simulink model "SMC_Lyapunov_PID_switch_com_m_change"  (R2016a)
settings: Solver=VariableStepAuto  StartTime=0.0  StopTime=50  RelTol=1e-3
libraries: simulink x2
settings Model: Creator=Jie WEN  LastModifiedBy=张涵

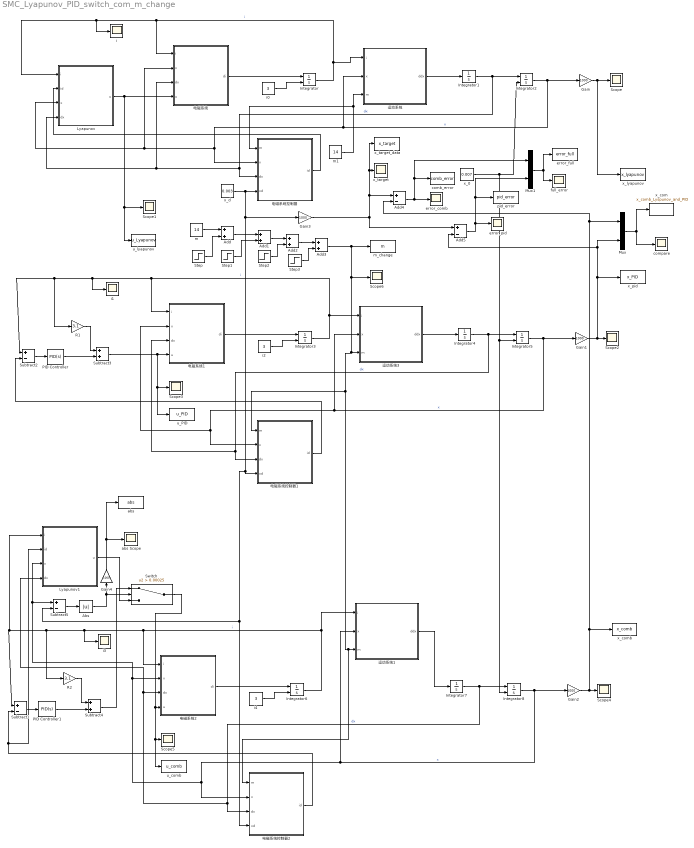
== system SMC_Lyapunov_PID_switch_com_m_change ==
  Abs : Abs
  Add{,1..3} (4 alike) : Sum
  Add4 : Sum  Inputs=+-
  Add5 : Sum  Inputs=+-
  Gain{,1..4} (5 alike) : Gain  Gain=1000
  Integrator : Integrator  InitialConditionSource=external  InitialCondition=3
  Integrator1 : Integrator
  Integrator2 : Integrator  InitialConditionSource=external  InitialCondition=7
  Integrator3 : Integrator  InitialConditionSource=external  InitialCondition=3
  Integrator4 : Integrator
  Integrator5 : Integrator  InitialConditionSource=external  InitialCondition=7
  Integrator6 : Integrator  InitialConditionSource=external  InitialCondition=3
  Integrator7 : Integrator
  Integrator8 : Integrator  InitialConditionSource=external  InitialCondition=7
  Lyapunov : MATLAB Function  TreatAsAtomicUnit=on
  Lyapunov1 : MATLAB Function  TreatAsAtomicUnit=on
  Mux : Mux  Inputs=2
  Mux1 : Mux  Inputs=2
  PID Controller : simulink/Continuous/PID Controller  Controller=PID  Form=Parallel  TimeDomain=Continuous-time  SampleTime=-1  IntegratorMethod=Forward Euler  ControllerParametersSource=internal  P=-6  I=0.1  D=0.1  UseFilter=on  N=100  InitialConditionSource=internal  InitialConditionForIntegrator=0  InitialConditionForFilter=0  DifferentiatorICPrevScaledInput=0  ExternalReset=none  TrackingMode=off  Kt=1  LimitOutput=off  UpperSaturationLimit=inf  LowerSaturationLimit=-inf  LinearizeAsGain=on  AntiWindupMode=none  Kb=1  POutMin=[]  POutMax=[]  IOutMin=[]  IOutMax=[]  DOutMin=[]  DOutMax=[]  NOutMin=[]  NOutMax=[]  SumOutMin=[]  SumOutMax=[]  SaturationOutMin=[]  SaturationOutMax=[]  PParamMin=[]  PParamMax=[]  IParamMin=[]  IParamMax=[]  DParamMin=[]  DParamMax=[]  NParamMin=[]  NParamMax=[]  KbParamMin=[]  KbParamMax=[]  KtParamMin=[]  KtParamMax=[]  KbOutMin=[]  KbOutMax=[]  KtOutMin=[]  KtOutMax=[]  IntegratorOutMin=[]  IntegratorOutMax=[]  FilterOutMin=[]  FilterOutMax=[]  SumI1OutMin=[]  SumI1OutMax=[]  SumI2OutMin=[]  SumI2OutMax=[]  SumI3OutMin=[]  SumI3OutMax=[]  SumDOutMin=[]  SumDOutMax=[]  DifferentiatorOutMin=[]  DifferentiatorOutMax=[]  IntegratorContinuousStateAttributes=''  IntegratorStateMustResolveToSignalObject=off  IntegratorRTWStateStorageClass=Auto  FilterContinuousStateAttributes=''  FilterStateMustResolveToSignalObject=off  FilterRTWStateStorageClass=Auto
  PID Controller1 : simulink/Continuous/PID Controller  Controller=PID  Form=Parallel  TimeDomain=Continuous-time  SampleTime=-1  IntegratorMethod=Forward Euler  ControllerParametersSource=internal  P=-6  I=0.1  D=0.1  UseFilter=on  N=100  InitialConditionSource=internal  InitialConditionForIntegrator=0  InitialConditionForFilter=0  DifferentiatorICPrevScaledInput=0  ExternalReset=none  TrackingMode=off  Kt=1  LimitOutput=off  UpperSaturationLimit=inf  LowerSaturationLimit=-inf  LinearizeAsGain=on  AntiWindupMode=none  Kb=1  POutMin=[]  POutMax=[]  IOutMin=[]  IOutMax=[]  DOutMin=[]  DOutMax=[]  NOutMin=[]  NOutMax=[]  SumOutMin=[]  SumOutMax=[]  SaturationOutMin=[]  SaturationOutMax=[]  PParamMin=[]  PParamMax=[]  IParamMin=[]  IParamMax=[]  DParamMin=[]  DParamMax=[]  NParamMin=[]  NParamMax=[]  KbParamMin=[]  KbParamMax=[]  KtParamMin=[]  KtParamMax=[]  KbOutMin=[]  KbOutMax=[]  KtOutMin=[]  KtOutMax=[]  IntegratorOutMin=[]  IntegratorOutMax=[]  FilterOutMin=[]  FilterOutMax=[]  SumI1OutMin=[]  SumI1OutMax=[]  SumI2OutMin=[]  SumI2OutMax=[]  SumI3OutMin=[]  SumI3OutMax=[]  SumDOutMin=[]  SumDOutMax=[]  DifferentiatorOutMin=[]  DifferentiatorOutMax=[]  IntegratorContinuousStateAttributes=''  IntegratorStateMustResolveToSignalObject=off  IntegratorRTWStateStorageClass=Auto  FilterContinuousStateAttributes=''  FilterStateMustResolveToSignalObject=off  FilterRTWStateStorageClass=Auto
  R1 : Gain  Gain=3.1
  R2 : Gain  Gain=3.1
  Scope{,1..6} (7 alike) : Scope
  Step : Step  Time=10  After=0.2  SampleTime=0
  Step1 : Step  Time=20  After=-0.2  SampleTime=0
  Step2 : Step  Time=30  After=-0.1  SampleTime=0
  Step3 : Step  Time=40  After=0.1  SampleTime=0
  Subtract1 : Sum  Inputs=+-
  Subtract2 : Sum  Inputs=+-
  Subtract3 : Sum
  Subtract4 : Sum
  Subtract5 : Sum  Inputs=+-
  Switch : Switch  Criteria=u2 > Threshold  Threshold=0.00025
  abs : ToWorkspace  VariableName=abs  SampleTime=-1
  abs Scope : Scope
  comb_error : ToWorkspace  VariableName=comb_error  SampleTime=-1
  compare : Scope
  error_comb : Scope
  error_full : ToWorkspace  VariableName=error_full  SampleTime=-1
  error_pid : Scope
  full_error : Scope
  i : Scope
  i0 : Constant  Value=3
  i1 : Scope
  i2 : Constant  Value=3
  i3 : Scope
  i4 : Constant  Value=3
  m : Constant  Value=14
  m1 : Constant  Value=14
  m_change : ToWorkspace  VariableName=m  SampleTime=-1
  pid_error : ToWorkspace  VariableName=pid_error  SampleTime=-1
  u_PID : ToWorkspace  VariableName=u_PID  SampleTime=-1
  u_comb : ToWorkspace  VariableName=u_comb  SampleTime=-1
  u_lyapunov : ToWorkspace  VariableName=u_Lyapunov  SampleTime=-1
  x_0 : Constant  Value=0.007
  x_com : ToWorkspace  VariableName=x_comb_Lyspunov_and_PID  SampleTime=-1
  x_comb : ToWorkspace  VariableName=x_comb  SampleTime=-1
  x_d : Constant  Value=0.003
  x_lyapunov : ToWorkspace  VariableName=x_lyapunov  SampleTime=-1
  x_pid : ToWorkspace  VariableName=x_PID  SampleTime=-1
  x_target : Scope
  x_target_data : ToWorkspace  VariableName=x_target  SampleTime=-1
  电磁系统 : MATLAB Function  TreatAsAtomicUnit=on
  电磁系统1 : MATLAB Function  TreatAsAtomicUnit=on
  电磁系统2 : MATLAB Function  TreatAsAtomicUnit=on
  电磁系统控制器 : MATLAB Function  TreatAsAtomicUnit=on
  电磁系统控制器1 : MATLAB Function  TreatAsAtomicUnit=on
  电磁系统控制器2 : MATLAB Function  TreatAsAtomicUnit=on
  运动系统 : MATLAB Function  TreatAsAtomicUnit=on
  运动系统1 : MATLAB Function  TreatAsAtomicUnit=on
  运动系统3 : MATLAB Function  TreatAsAtomicUnit=on
  wires:
  电磁系统/1(di) -> Integrator/1
  运动系统/1(ddx) -> Integrator1/1
  Integrator1/1 -> Lyapunov/4(dx), 电磁系统/3(dx), 电磁系统控制器/3(dx), Integrator2/1  "dx"
  Integrator2/1 -> Gain/1, Lyapunov/3(x), 电磁系统/2(x), 电磁系统控制器/2(x), 运动系统/2(x)  "x"
  Integrator/1 -> 运动系统/1(i), 电磁系统/1(i), Lyapunov/1(i), i/1  "i"
  电磁系统控制器/1(id) -> Lyapunov/2(id)
  Gain/1 -> x_lyapunov/1, Scope/1
  Lyapunov/1(u) -> u_lyapunov/1, Scope1/1, 电磁系统/4(u)
  i0/1 -> Integrator/2
  电磁系统1/1(di) -> Integrator3/1
  运动系统3/1(ddx) -> Integrator4/1
  Integrator4/1 -> 电磁系统1/3(dx), 电磁系统控制器1/3(dx), Integrator5/1  "dx"
  Integrator5/1 -> Gain1/1, 运动系统3/2(x), 电磁系统控制器1/2(x), 电磁系统1/2(x)  "x"
  Integrator3/1 -> 运动系统3/1(i), 电磁系统1/1(i), i1/1, R1/1, Subtract2/1  "i"
  电磁系统控制器1/1(id) -> Subtract2/2
  Subtract2/1 -> PID Controller/1
  PID Controller/1 -> Subtract3/2
  R1/1 -> Subtract3/1
  Subtract3/1 -> u_PID/1, Scope3/1, 电磁系统1/4(u)
  i2/1 -> Integrator3/2
  Mux/1 -> x_com/1, compare/1
  Integrator8/1 -> Gain2/1, 运动系统1/2(x), 电磁系统控制器2/2(x), 电磁系统2/2(x), Subtract5/1, Lyapunov1/3(x)  "x"
  i4/1 -> Integrator6/2
  Integrator7/1 -> Lyapunov1/4(dx), 电磁系统2/3(dx), 电磁系统控制器2/3(dx), Integrator8/1  "dx"
  x_0/1 -> Integrator2/2, Integrator8/2, Integrator5/2
  电磁系统控制器2/1(id) -> Lyapunov1/2(id), Subtract1/2
  x_d/1 -> Subtract5/2, 电磁系统控制器2/4(xd), 电磁系统控制器1/4(xd), Gain3/1, 电磁系统控制器/4(xd)
  运动系统1/1(ddx) -> Integrator7/1
  Subtract1/1 -> PID Controller1/1
  R2/1 -> Subtract4/1
  Subtract4/1 -> Switch/1
  PID Controller1/1 -> Subtract4/2
  Integrator6/1 -> 运动系统1/1(i), 电磁系统2/1(i), i3/1, R2/1, Lyapunov1/1(i), Subtract1/1  "i"
  电磁系统2/1(di) -> Integrator6/1
  Switch/1 -> u_comb/1, Scope5/1, 电磁系统2/4(u)
  Subtract5/1 -> Abs/1
  Abs/1 -> Gain4/1, Switch/2
  Lyapunov1/1(u) -> Switch/3
  m/1 -> Add/1
  Step/1 -> Add/2
  m1/1 -> 运动系统/3(m), 电磁系统控制器/1(m)
  Step1/1 -> Add1/2
  Add/1 -> Add1/1
  Add1/1 -> Add2/1
  Step2/1 -> Add2/2
  Add2/1 -> Add3/1
  Step3/1 -> Add3/2
  Add3/1 -> Scope6/1, 电磁系统控制器1/1(m), 电磁系统控制器2/1(m), 运动系统1/3(m), 运动系统3/3(m), m_change/1
  Gain3/1 -> Add4/1, x_target/1, x_target_data/1, Add5/1
  Gain1/1 -> Add5/2, Mux/2, x_pid/1, Scope2/1
  Gain2/1 -> Add4/2, Mux/1, x_comb/1, Scope4/1
  Add4/1 -> Mux1/1, comb_error/1, error_comb/1
  Add5/1 -> Mux1/2, pid_error/1, error_pid/1
  Mux1/1 -> full_error/1, error_full/1
  Gain4/1 -> abs/1, abs Scope/1

== matlab function SMC_Lyapunov_PID_switch_com_m_change/运动系统 ==
  data: i input; ddx output; x input; m input
function ddx = fcn(i,x,m)
% m=14;
g=9.8;
C=7.8e-4;
ddx=g-(C/m)*(i^2/x^2);

== matlab function SMC_Lyapunov_PID_switch_com_m_change/电磁系统 ==
  data: i input; x input; dx input; u input; di output
function di = fcn(i,x,dx,u)
%#codegen
R=3.1;
C=7.8e-4;
di=(u-R*i+2*C*i*dx/x^2)*x/(2*C);

== matlab function SMC_Lyapunov_PID_switch_com_m_change/电磁系统控制器 ==
  data: m input; x input; dx input; xd input; id output
function id = fcn(m,x,dx,xd)
% m=14;
g=9.8;
C=7.8e-4;
x2=dx;
p11=0.2;
p22=p11;
x1=x;
pp=0.00001;
if (x1-xd)*x2>0
    p12=pp;
else
    p12=-pp;
end
p21=p12;
P=[p11 p12;
   p21 p22];
k_lya1=1;
G=(p11*x2+p21*g+p11*(x1-xd)+p21*x2+p12*x2)*(x1-xd)+(p12*x2+p22*g+p22*x2)*x2;
F=(C*p21*(x1-xd)+C*p22*x2)/(m*x1^2)
double_i=G/F+k_lya1*F;
id=sqrt(abs(double_i));

== matlab function SMC_Lyapunov_PID_switch_com_m_change/电磁系统1 ==
  data: i input; x input; dx input; u input; di output
function di = fcn(i,x,dx,u)
%#codegen
R=3.1;
C=7.8e-4;
di=(u-R*i+2*C*i*dx/x^2)*x/(2*C);

== matlab function SMC_Lyapunov_PID_switch_com_m_change/电磁系统控制器1 ==
  data: m input; x input; dx input; xd input; id output
function id = fcn(m,x,dx,xd)
% m=14;
g=9.8;
C=7.8e-4;
x2=dx;
c1=1.5;
k1=10;
c2=0.001;
s=c1*(x-xd)+dx;
double_i=m*x^2/C*(c1*x2+g+k1*s+c2*sign(s));
id=sqrt(abs(double_i));

== matlab function SMC_Lyapunov_PID_switch_com_m_change/运动系统1 ==
  data: i input; ddx output; x input; m input
function ddx = fcn(i,x,m)
% m=14;
g=9.8;
C=7.8e-4;
ddx=g-(C/m)*(i^2/x^2);

== matlab function SMC_Lyapunov_PID_switch_com_m_change/Lyapunov ==
  data: i input; id input; x input; dx input; u output
function u = fcn(i,id,x,dx)
%#codegen
R=3.1;
C=7.8e-4;
%k=1.25;
k=2;
u=(R-(2*C*dx/x))*i-k*(i-id)*x/(2*C);

== matlab function SMC_Lyapunov_PID_switch_com_m_change/电磁系统2 ==
  data: i input; x input; dx input; u input; di output
function di = fcn(i,x,dx,u)
%#codegen
R=3.1;
C=7.8e-4;
di=(u-R*i+2*C*i*dx/x^2)*x/(2*C);

== matlab function SMC_Lyapunov_PID_switch_com_m_change/电磁系统控制器2 ==
  data: m input; x input; dx input; xd input; id output
function id = fcn(m,x,dx,xd)
% m=14;
g=9.8;
C=7.8e-4;
x2=dx;
c1=1.5;
k1=10;
c2=0.001;
s=c1*(x-xd)+dx;
double_i=m*x^2/C*(c1*x2+g+k1*s+c2*sign(s));
id=sqrt(abs(double_i));

== matlab function SMC_Lyapunov_PID_switch_com_m_change/Lyapunov1 ==
  data: i input; id input; x input; dx input; u output
function u = fcn(i,id,x,dx)
%#codegen
R=3.1;
C=7.8e-4;
%k=1.25;
k=2;
u=(R-(2*C*dx/x))*i-k*(i-id)*x/(2*C);

== matlab function SMC_Lyapunov_PID_switch_com_m_change/运动系统3 ==
  data: i input; ddx output; x input; m input
function ddx = fcn(i,x,m)
% m=14;
g=9.8;
C=7.8e-4;
ddx=g-(C/m)*(i^2/x^2);
